simulink model "controllo_motori"  (R2025b)
settings: Solver=FixedStepAuto  StartTime=0.0  StopTime=10  FixedStep=0.01  RelTol=1e-3
libraries: slpidlib x3, vehdynlibtire x2, simulink x2, vehdynlibsteering x1, autolibshared x1
(part 1 of 2)
settings Model: SimulationMode=accelerator  Creator=lori2  LastModifiedBy=zinga

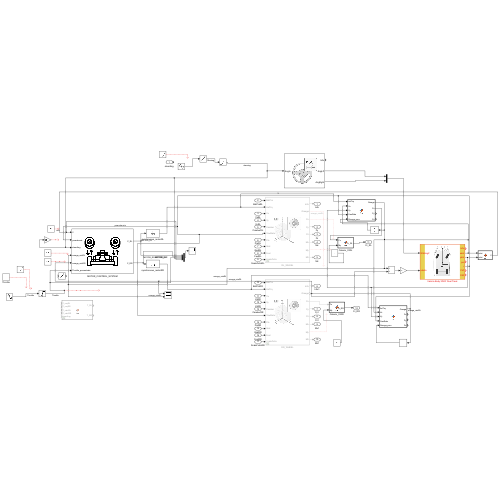
[thumbnail: Simulink's stored preview of the top-level diagram]
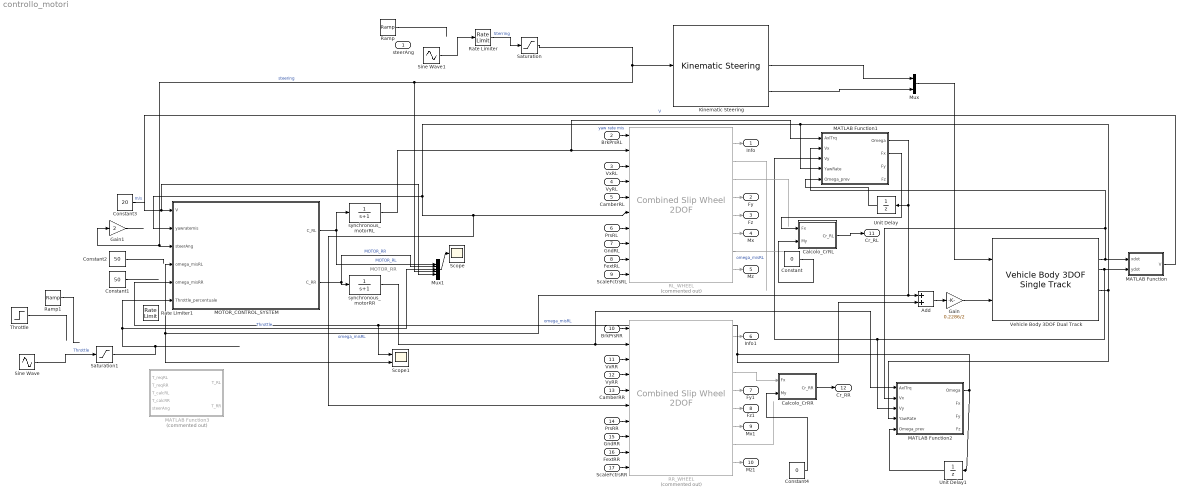
== system controllo_motori ==
  note: MOTOR_RR
  steerAng : Inport
  BrkPrsRL : Inport  Port=2
  VxRL : Inport  Port=3
  VyRL : Inport  Port=4
  CamberRL : Inport  Port=5
  PrsRL : Inport  Port=6
  GndRL : Inport  Port=7
  FextRL : Inport  Port=8
  ScaleFctrsRL : Inport  Port=9
  BrkPrsRR : Inport  Port=10
  VxRR : Inport  Port=11
  VyRR : Inport  Port=12
  CamberRR : Inport  Port=13
  PrsRR : Inport  Port=14
  GndRR : Inport  Port=15
  FextRR : Inport  Port=16
  ScaleFctrsRR : Inport  Port=17
  Add : Sum
  Calcolo_CrRL : MATLAB Function  TreatAsAtomicUnit=on
  Calcolo_CrRR : MATLAB Function  TreatAsAtomicUnit=on
  Constant : Constant  Value=0
  Constant1 : Constant  Value=50
  Constant2 : Constant  Value=50
  Constant3 : Constant  Value=20
  Constant4 : Constant  Value=0
  Gain : Gain  Gain=0.2286/2
  Gain1 : Gain  Gain=2
  Kinematic Steering : vehdynlibsteering/Kinematic Steering  StrgType=Ackerman  StrgRatioType=Constant  Loc=Front  NrmlFctr=0.01  TrckWdth=1.2  WhlBase=0.336  Db=0  StrgRng=1.25*pi  StrgAngBpts="[-6.2832   -5.0265   -3.7699   -2.5133   -1.2566         0    1.2566    2.5133    3.7699    5.0265    6.2832]"  StrgRatioTbl=|  StrgRatio=100  PctAckIn=off  PctAck=100  PctAckTbl=ones(1,11)*100  StrgArmLngth=0.1  RckCsLngth=0.5  TieRodLngth=0.248  D=0.2  PnnRadius=0.00085818  PnnRadiusTbl="[0.0055    0.0055    0.0056    0.0057    0.0058    0.0057    0.0057    0.0057    0.0056    0.0055    0.0055]"  RodLngth=0.1  ParaArmLngth=0.9  aMode=2
      | [13.5000   13.3750   13.2500   13.1250   13.0000   13.0000   13.0000   13.1250   13.2500   13.3750   13.5000
      | ]
  MATLAB Function : MATLAB Function  TreatAsAtomicUnit=on
  MATLAB Function1 : MATLAB Function  TreatAsAtomicUnit=on
  MATLAB Function2 : MATLAB Function  TreatAsAtomicUnit=on
  MATLAB Function3 : MATLAB Function  Commented=on  TreatAsAtomicUnit=on
  MOTOR_CONTROL_SYSTEM : Subsystem
      mask Display: image('car_16221049.png', [0,0,0,0,80,80]);
  Mux : Mux  Inputs=2
  Mux1 : Mux  Inputs=5
  RL_WHEEL : vehdynlibtire/Combined Slip Wheel 2DOF  Commented=on  tireType=External file  tireParamSet=vdynPassCar.mat  vertType=Magic Formula  plySteer=on  turnslip=on  BrakeType=Disc  mu_static=.3  mu_kinetic=.2  drum_abore=0.0508  drum_a=0.123  drum_c=0.212  drum_r=0.15  drum_theta1=0  drum_theta2=126  disk_abore=.05  Rm=.177  num_pads=2  brake_p_bpt=[1 11.4736842105263 21.9473684210526 32.4210526315789 42.8947368421053 53.3684210526316 63.8421052631579 74.3157894736842 84.7894736842105 95.2631578947368 105.736842105263 116.210526315789 126.684210526316 137.157894736842 147.631578947368 158.105263157895 168.578947368421 179.052631578947 189.526315789474 200]  brake_n_bpt=[0 52.6315789473684 105.263157894737 157.894736842105 210.526315789474 263.157894736842 315.789473684211 368.421052631579 421.052631578947 473.684210526316 526.315789473684 578.947368421053 631.578947368421 684.210526315789 736.842105263158 789.473684210526 842.105263157895 894.736842105263 947.368421052632 1000]  f_brake_t=[43.4900602404453 42.5056030554862 41.5350898940194 40.5780454442085 39.6340111501808 38.7025443887544 37.7832176914519 36.8756180088306 35.9793460143796 35.0940154454303 34.2192524787115 33.3546951383474 32.4999927342521 31.6548053290159 30.8188032315107 29.991666515561 29.1730845621415 28.362755623661 27.5603864089927 26.765691687993;498.991217495636 487.695866636631 476.560505099801 465.579679307235 454.748127933653 444.060772460445 433.51270824929 423.099196101319 412.81565427025 402.657650900201 392.620896861006 382.701238955775 372.894653477208 363.197240090814 353.605216024701 344.114910546964 334.722759712992 325.425301366216 316.219170376863 307.10109410434;954.492374750826 932.886130217776 911.585920305583 890.581313170261 869.862244717126 849.419000532136 829.242198807128 809.322774193808 789.651962526121 770.221286354971 751.0225412433 732.047782773203 713.289314220164 694.739674852612 676.391628817892 658.238154578366 640.272434863842 622.48784710877 604.877954344734 587.436496520688;1409.99353200602 1378.07639379892 1346.61133551136 1315.58294703329 1284.9763615006 1254.77722860383 1224.97168936497 1195.5463522863 1166.48827078199 1137.78492180974 1109.42418562559 1081.39432659063 1053.68397496312 1026.28210961441 999.178041611083 972.361398609768 945.822110014692 919.550392851325 893.536738312604 867.771898937035;1865.49468926121 1823.26665738007 1781.63675071715 1740.58458089631 1700.09047828407 1660.13545667552 1620.7011799228 1581.76993037878 1543.32457903786 1505.34855726451 1467.82583000789 1430.74087040806 1394.07863570608 1357.82454437621 1321.96445440427 1286.48464264117 1251.37178516554 1216.61293859388 1182.19552228048 1148.10730135338;2320.9958465164 2268.45692096121 2216.66216592293 2165.58621475934 2115.20459506754 2065.49368474721 2016.43067048064 1967.99350847127 1920.16088729373 1872.91219271928 1826.22747439018 1780.08741422549 1734.47329644903 1689.36697913801 1644.75086719747 1600.60788667257 1556.92146031639 1513.67548433643 1470.85430624835 1428.44270376973;2776.49700377159 2713.64718454235 2651.68758112871 2590.58784862237 2530.31871185102 2470.8519128189 2412.16016103848 2354.21708656376 2296.9971955496 2240.47582817405 2184.62911877248 2129.43395804292 2074.86795719199 2020.9094138998 1967.53727999066 1914.73113070398 1862.47113546724 1810.73803007899 1759.51309021622 1708.77810618608;3231.99816102678 3158.8374481235 3086.71299633449 3015.58948248539 2945.43282863449 2876.21014089059 2807.88965159632 2740.44066465625 2673.83350380547 2608.03946362882 2543.03076315477 2478.78050186034 2415.26261793494 2352.4518486616 2290.32369278385 2228.85437473538 2168.02081061809 2107.80057582154 2048.17187418409 1989.11350860242;3687.49931828197 3604.02771170464 3521.73841154027 3440.59111634842 3360.54694541796 3281.56836896228 3203.61914215416 3126.66424274874 3050.66981206134 2975.60309908359 2901.43240753707 2828.12704567777 2755.6572786779 2683.9942834234 2613.11010557704 2542.97761876678 2473.57048576894 2404.8631215641 2336.83065815196 2269.44891101877;4143.00047553716 4049.21797528579 3956.76382674606 3865.59275021144 3775.66106220143 3686.92659703397 3599.34863271199 3512.88782084123 3427.50612031721 3343.16673453836 3259.83405191936 3177.4735894952 3096.05193942085 3015.5367181852 2935.89651837023 2857.10086279818 2779.12016091979 2701.92566730665 2625.48944211983 2549.78431343512;4598.50163279235 4494.40823886693 4391.78924195184 4290.59438407447 4190.77517898491 4092.28482510566 3995.07812326983 3899.11139893372 3804.34242857308 3710.73036999313 3618.23569630166 3526.82013331263 3436.44660016381 3347.079152947 3258.68293116342 3171.22410682959 3084.66983607064 2998.98821304921 2914.1482260877 2830.11971585147;5054.00279004754 4939.59850244808 4826.81465715762 4715.59601793749 4605.88929576838 4497.64305317735 4390.80761382767 4285.3349770262 4181.17873682896 4078.2940054479 3976.63734068395 3876.16667713006 3776.84126090677 3678.62158770879 3581.46934395661 3485.34735086099 ...(+2764 chars)]  NOMPRES=262000  PRESMAX=1000000  PRESMIN=10000  FNOMIN=4300  FZMAX=8600  FZMIN=100  VXLOW=1  KPUMAX=1.5  KPUMIN=-1.5  ALPMAX=1.5  ALPMIN=-1.5  CAMMAX=0.17453  CAMMIN=-0.17453  LONGVL=16.7  FxRelFreqLwrLim=200*pi  FyRelFreqLwrLim=200*pi  MyRelFreqLwrLim=100*pi  omegao=0  UNLOADED_RADIUS=0.33454  WIDTH=0.235  RIM_RADIUS=0.2286  ASPECT_RATIO=0.45  MASS=11.2  IYY=1.084  br=1e-3  GRAVITY=-9.81  zo=0  zdoto=0  BREFF=8.25094594147963  DREFF=0.260468730454265  FREFF=0.0735298544471851  Q_RE0=1.00866439868088  Q_V1=0.000760413786224011  Q_V2=0.0463384792019201  Q_FZ1=0  Q_FZ2=15.6870832810226  Q_FZ3=0  Q_FCX=0.138643970247602  Q_FCY=0.10843499565426  Q_FCY2=-0.465763352339538  PFZ1=0.69958166705601  VERTICAL_STIFFNESS=207885.061134007  VERTICAL_DAMPING=500  BOTTOM_OFFST=0.00990653336182505  BOTTOM_STIFF=1999075.87051971  Q_CAM1=86.7791723017291  Q_CAM2=259.705254231766  Q_CAM3=0.510281667378416  Q_FYS1=-20769.4728880343  Q_FYS2=-59060.183485617  Q_FYS3=89271.8260126986  LONGITUDINAL_STIFFNESS=388714.175879854  LATERAL_STIFFNESS=157087.404633332  PCFX1=0.18539229191199  PCFX2=0  PCFX3=0  PCFY1=0.163183345037677  PCFY2=0  PCFY3=0.249094918231954  Q_RA1=0.675942571700787  Q_RA2=0.73800463546164  Q_RB1=1.04487486456705  Q_RB2=-1.191763806629  PCX1=1.58523057950359  PDX1=1.0239116238178  PDX2=-0.0842405110022724  PDX3=0  PEX1=0.110312777158455  PEX2=0.313468516038146  PEX3=0  PEX4=0.0016060905760045  PKX1=21.3872544684023  PKX2=14.0006541873175  PKX3=-0.405326109653452  PHX1=0.000212599305364818  PHX2=0.00115950515263055  PVX1=1.59236164471432e-05  PVX2=0.000104321112127671  PPX1=-0.349461321276586  PPX2=0.387840040616429  PPX3=-0.0969947336569324  PPX4=0.0632271859795801  RBX1=12.7633329850276  RBX2=9.5787123658471  RBX3=0  RCX1=1.02796280922059  REX1=-0.45202516851367  REX2=-0.47304886171176  RHX1=0.000233272373115809  QSX1=-0.00788307788961443  QSX2=0.954629515459396  QSX3=0.0155855777667025  QSX4=0.125904607142414  QSX5=1.01110069703963  QSX6=20.1938577118433  QSX7=0.310818120717083  QSX8=-0.0430823751139655  QSX9=0.636494404888216  QSX10=0.142438060591663  QSX11=0.346766530036373  QSX12=0  QSX13=0  QSX14=0  PPMX1=0  PCY1=1.34299950037631  PDY1=0.878267729082195  PDY2=-0.0644597923147385  PDY3=0  PEY1=-0.809776534470972  PEY2=-0.600180598867198  PEY3=0.0991732552633487  PEY4=-6.5577974035573  PEY5=0  PKY1=-15.5714726518315  PKY2=1.73126522291751  PKY3=0.365349873517229  PKY4=1.98176755955416  PKY5=0  PKY6=-0.884005199550313  PKY7=-0.237259727611847  PHY1=-0.00183370557235628  PHY2=0.00346401302716671  PVY1=-0.00675427560163264  PVY2=0.036379218103843  PVY3=-0.163543984089166  PVY4=-0.491003349625726  PPY1=-0.62059646553185  PPY2=-0.0647824842338686  PPY3=-0.164648843290686  PPY4=0.283193909060098  PPY5=0  RBY1=10.7588809173639  RBY2=7.70420065295029  RBY3=3.40283755070691e-06  RBY4=0  RCY1=1.06691874059059  REY1=0.308244924574305  REY2=7.48775032604508e-06  RHY1=0.0118479204960415  RHY2=7.63650177161071e-06  RVY1=0.0560024425050078  RVY2=7.48487127056197e-06  RVY3=0  RVY4=98.4047026517149  RVY5=2.02759273900054  RVY6=15.7623064923347  QSY1=0.00699077564863536  QSY2=0  QSY3=0.00153535478298811  QSY4=8.55710322455322e-05  QSY5=0  QSY6=0  QSY7=0.89443879773793  QSY8=-0.403227641260894  QBZ1=11.666656027484  QBZ2=-1.30355438574485  QBZ3=0  QBZ4=0.177918305399071  QBZ5=-0.162481135068033  QBZ6=0  QBZ9=30.1445534682089  QBZ10=0  QCZ1=1.29026978207574  QDZ1=0.0886972644991399  QDZ2=-0.0058634820161856  QDZ3=0.3805597481383  QDZ4=0  QDZ6=0.00160914918118959  QDZ7=-0.00211036330862154  QDZ8=-0.13921904912557  QDZ9=0.00816585550028243  QDZ10=0  QDZ11=0  QEZ1=-2.19802254534746  QEZ2=1.01850535789165  QEZ3=0  QEZ4=0.278379679112054  QEZ5=-0.548414722765386  QHZ1=0.00148361198869669  QHZ2=0.00202017567585904  QHZ3=0.240316641332066  QHZ4=-0.210114035738085  PPZ1=-0.443927982388615  PPZ2=0  SSZ1=0.00914999585397887  SSZ2=0.0389830656052735  SSZ3=0  SSZ4=0  PDXP1=0.396718274678791  PDXP2=0  PDXP3=0  PKYP1=1.00587060633573  PDYP1=0.40483048923438  PDYP2=0  PDYP3=0  PDYP4=0  PHYP1=0.992731942067188  PHYP2=0.150352945499914  PHYP3=0  PHYP4=-3.98988682633674  PECP1=0.502379254513503  PECP2=0  QDTP1=10.0178654287947  QCRP1=0.200627747200702  QCRP2=0.0995735881599772  QBRP1=0.0997107127960717  QDRP1=1.01432910167423  QDRP2=0  aMode=2
  RR_WHEEL : vehdynlibtire/Combined Slip Wheel 2DOF  Commented=on  tireType=External file  tireParamSet=vdynPassCar.mat  vertType=Magic Formula  plySteer=on  turnslip=on  BrakeType=Disc  mu_static=.3  mu_kinetic=.2  drum_abore=0.0508  drum_a=0.123  drum_c=0.212  drum_r=0.15  drum_theta1=0  drum_theta2=126  disk_abore=.05  Rm=.177  num_pads=2  brake_p_bpt=[1 11.4736842105263 21.9473684210526 32.4210526315789 42.8947368421053 53.3684210526316 63.8421052631579 74.3157894736842 84.7894736842105 95.2631578947368 105.736842105263 116.210526315789 126.684210526316 137.157894736842 147.631578947368 158.105263157895 168.578947368421 179.052631578947 189.526315789474 200]  brake_n_bpt=[0 52.6315789473684 105.263157894737 157.894736842105 210.526315789474 263.157894736842 315.789473684211 368.421052631579 421.052631578947 473.684210526316 526.315789473684 578.947368421053 631.578947368421 684.210526315789 736.842105263158 789.473684210526 842.105263157895 894.736842105263 947.368421052632 1000]  f_brake_t=[43.4900602404453 42.5056030554862 41.5350898940194 40.5780454442085 39.6340111501808 38.7025443887544 37.7832176914519 36.8756180088306 35.9793460143796 35.0940154454303 34.2192524787115 33.3546951383474 32.4999927342521 31.6548053290159 30.8188032315107 29.991666515561 29.1730845621415 28.362755623661 27.5603864089927 26.765691687993;498.991217495636 487.695866636631 476.560505099801 465.579679307235 454.748127933653 444.060772460445 433.51270824929 423.099196101319 412.81565427025 402.657650900201 392.620896861006 382.701238955775 372.894653477208 363.197240090814 353.605216024701 344.114910546964 334.722759712992 325.425301366216 316.219170376863 307.10109410434;954.492374750826 932.886130217776 911.585920305583 890.581313170261 869.862244717126 849.419000532136 829.242198807128 809.322774193808 789.651962526121 770.221286354971 751.0225412433 732.047782773203 713.289314220164 694.739674852612 676.391628817892 658.238154578366 640.272434863842 622.48784710877 604.877954344734 587.436496520688;1409.99353200602 1378.07639379892 1346.61133551136 1315.58294703329 1284.9763615006 1254.77722860383 1224.97168936497 1195.5463522863 1166.48827078199 1137.78492180974 1109.42418562559 1081.39432659063 1053.68397496312 1026.28210961441 999.178041611083 972.361398609768 945.822110014692 919.550392851325 893.536738312604 867.771898937035;1865.49468926121 1823.26665738007 1781.63675071715 1740.58458089631 1700.09047828407 1660.13545667552 1620.7011799228 1581.76993037878 1543.32457903786 1505.34855726451 1467.82583000789 1430.74087040806 1394.07863570608 1357.82454437621 1321.96445440427 1286.48464264117 1251.37178516554 1216.61293859388 1182.19552228048 1148.10730135338;2320.9958465164 2268.45692096121 2216.66216592293 2165.58621475934 2115.20459506754 2065.49368474721 2016.43067048064 1967.99350847127 1920.16088729373 1872.91219271928 1826.22747439018 1780.08741422549 1734.47329644903 1689.36697913801 1644.75086719747 1600.60788667257 1556.92146031639 1513.67548433643 1470.85430624835 1428.44270376973;2776.49700377159 2713.64718454235 2651.68758112871 2590.58784862237 2530.31871185102 2470.8519128189 2412.16016103848 2354.21708656376 2296.9971955496 2240.47582817405 2184.62911877248 2129.43395804292 2074.86795719199 2020.9094138998 1967.53727999066 1914.73113070398 1862.47113546724 1810.73803007899 1759.51309021622 1708.77810618608;3231.99816102678 3158.8374481235 3086.71299633449 3015.58948248539 2945.43282863449 2876.21014089059 2807.88965159632 2740.44066465625 2673.83350380547 2608.03946362882 2543.03076315477 2478.78050186034 2415.26261793494 2352.4518486616 2290.32369278385 2228.85437473538 2168.02081061809 2107.80057582154 2048.17187418409 1989.11350860242;3687.49931828197 3604.02771170464 3521.73841154027 3440.59111634842 3360.54694541796 3281.56836896228 3203.61914215416 3126.66424274874 3050.66981206134 2975.60309908359 2901.43240753707 2828.12704567777 2755.6572786779 2683.9942834234 2613.11010557704 2542.97761876678 2473.57048576894 2404.8631215641 2336.83065815196 2269.44891101877;4143.00047553716 4049.21797528579 3956.76382674606 3865.59275021144 3775.66106220143 3686.92659703397 3599.34863271199 3512.88782084123 3427.50612031721 3343.16673453836 3259.83405191936 3177.4735894952 3096.05193942085 3015.5367181852 2935.89651837023 2857.10086279818 2779.12016091979 2701.92566730665 2625.48944211983 2549.78431343512;4598.50163279235 4494.40823886693 4391.78924195184 4290.59438407447 4190.77517898491 4092.28482510566 3995.07812326983 3899.11139893372 3804.34242857308 3710.73036999313 3618.23569630166 3526.82013331263 3436.44660016381 3347.079152947 3258.68293116342 3171.22410682959 3084.66983607064 2998.98821304921 2914.1482260877 2830.11971585147;5054.00279004754 4939.59850244808 4826.81465715762 4715.59601793749 4605.88929576838 4497.64305317735 4390.80761382767 4285.3349770262 4181.17873682896 4078.2940054479 3976.63734068395 3876.16667713006 3776.84126090677 3678.62158770879 3581.46934395661 3485.34735086099 ...(+2764 chars)]  NOMPRES=262000  PRESMAX=1000000  PRESMIN=10000  FNOMIN=4300  FZMAX=8600  FZMIN=100  VXLOW=1  KPUMAX=1.5  KPUMIN=-1.5  ALPMAX=1.5  ALPMIN=-1.5  CAMMAX=0.17453  CAMMIN=-0.17453  LONGVL=16.7  FxRelFreqLwrLim=200*pi  FyRelFreqLwrLim=200*pi  MyRelFreqLwrLim=100*pi  omegao=0  UNLOADED_RADIUS=0.33454  WIDTH=0.235  RIM_RADIUS=0.2286  ASPECT_RATIO=0.45  MASS=11.2  IYY=1.084  br=1e-3  GRAVITY=-9.81  zo=0  zdoto=0  BREFF=8.25094594147963  DREFF=0.260468730454265  FREFF=0.0735298544471851  Q_RE0=1.00866439868088  Q_V1=0.000760413786224011  Q_V2=0.0463384792019201  Q_FZ1=0  Q_FZ2=15.6870832810226  Q_FZ3=0  Q_FCX=0.138643970247602  Q_FCY=0.10843499565426  Q_FCY2=-0.465763352339538  PFZ1=0.69958166705601  VERTICAL_STIFFNESS=207885.061134007  VERTICAL_DAMPING=500  BOTTOM_OFFST=0.00990653336182505  BOTTOM_STIFF=1999075.87051971  Q_CAM1=86.7791723017291  Q_CAM2=259.705254231766  Q_CAM3=0.510281667378416  Q_FYS1=-20769.4728880343  Q_FYS2=-59060.183485617  Q_FYS3=89271.8260126986  LONGITUDINAL_STIFFNESS=388714.175879854  LATERAL_STIFFNESS=157087.404633332  PCFX1=0.18539229191199  PCFX2=0  PCFX3=0  PCFY1=0.163183345037677  PCFY2=0  PCFY3=0.249094918231954  Q_RA1=0.675942571700787  Q_RA2=0.73800463546164  Q_RB1=1.04487486456705  Q_RB2=-1.191763806629  PCX1=1.58523057950359  PDX1=1.0239116238178  PDX2=-0.0842405110022724  PDX3=0  PEX1=0.110312777158455  PEX2=0.313468516038146  PEX3=0  PEX4=0.0016060905760045  PKX1=21.3872544684023  PKX2=14.0006541873175  PKX3=-0.405326109653452  PHX1=0.000212599305364818  PHX2=0.00115950515263055  PVX1=1.59236164471432e-05  PVX2=0.000104321112127671  PPX1=-0.349461321276586  PPX2=0.387840040616429  PPX3=-0.0969947336569324  PPX4=0.0632271859795801  RBX1=12.7633329850276  RBX2=9.5787123658471  RBX3=0  RCX1=1.02796280922059  REX1=-0.45202516851367  REX2=-0.47304886171176  RHX1=0.000233272373115809  QSX1=-0.00788307788961443  QSX2=0.954629515459396  QSX3=0.0155855777667025  QSX4=0.125904607142414  QSX5=1.01110069703963  QSX6=20.1938577118433  QSX7=0.310818120717083  QSX8=-0.0430823751139655  QSX9=0.636494404888216  QSX10=0.142438060591663  QSX11=0.346766530036373  QSX12=0  QSX13=0  QSX14=0  PPMX1=0  PCY1=1.34299950037631  PDY1=0.878267729082195  PDY2=-0.0644597923147385  PDY3=0  PEY1=-0.809776534470972  PEY2=-0.600180598867198  PEY3=0.0991732552633487  PEY4=-6.5577974035573  PEY5=0  PKY1=-15.5714726518315  PKY2=1.73126522291751  PKY3=0.365349873517229  PKY4=1.98176755955416  PKY5=0  PKY6=-0.884005199550313  PKY7=-0.237259727611847  PHY1=-0.00183370557235628  PHY2=0.00346401302716671  PVY1=-0.00675427560163264  PVY2=0.036379218103843  PVY3=-0.163543984089166  PVY4=-0.491003349625726  PPY1=-0.62059646553185  PPY2=-0.0647824842338686  PPY3=-0.164648843290686  PPY4=0.283193909060098  PPY5=0  RBY1=10.7588809173639  RBY2=7.70420065295029  RBY3=3.40283755070691e-06  RBY4=0  RCY1=1.06691874059059  REY1=0.308244924574305  REY2=7.48775032604508e-06  RHY1=0.0118479204960415  RHY2=7.63650177161071e-06  RVY1=0.0560024425050078  RVY2=7.48487127056197e-06  RVY3=0  RVY4=98.4047026517149  RVY5=2.02759273900054  RVY6=15.7623064923347  QSY1=0.00699077564863536  QSY2=0  QSY3=0.00153535478298811  QSY4=8.55710322455322e-05  QSY5=0  QSY6=0  QSY7=0.89443879773793  QSY8=-0.403227641260894  QBZ1=11.666656027484  QBZ2=-1.30355438574485  QBZ3=0  QBZ4=0.177918305399071  QBZ5=-0.162481135068033  QBZ6=0  QBZ9=30.1445534682089  QBZ10=0  QCZ1=1.29026978207574  QDZ1=0.0886972644991399  QDZ2=-0.0058634820161856  QDZ3=0.3805597481383  QDZ4=0  QDZ6=0.00160914918118959  QDZ7=-0.00211036330862154  QDZ8=-0.13921904912557  QDZ9=0.00816585550028243  QDZ10=0  QDZ11=0  QEZ1=-2.19802254534746  QEZ2=1.01850535789165  QEZ3=0  QEZ4=0.278379679112054  QEZ5=-0.548414722765386  QHZ1=0.00148361198869669  QHZ2=0.00202017567585904  QHZ3=0.240316641332066  QHZ4=-0.210114035738085  PPZ1=-0.443927982388615  PPZ2=0  SSZ1=0.00914999585397887  SSZ2=0.0389830656052735  SSZ3=0  SSZ4=0  PDXP1=0.396718274678791  PDXP2=0  PDXP3=0  PKYP1=1.00587060633573  PDYP1=0.40483048923438  PDYP2=0  PDYP3=0  PDYP4=0  PHYP1=0.992731942067188  PHYP2=0.150352945499914  PHYP3=0  PHYP4=-3.98988682633674  PECP1=0.502379254513503  PECP2=0  QDTP1=10.0178654287947  QCRP1=0.200627747200702  QCRP2=0.0995735881599772  QBRP1=0.0997107127960717  QDRP1=1.01432910167423  QDRP2=0  aMode=2
  Ramp : simulink/Sources/Ramp  slope=-20  start=3  InitialOutput=0
  Ramp1 : simulink/Sources/Ramp  slope=10  start=0  InitialOutput=0
  Rate Limiter : RateLimiter  RisingSlewLimit=20  FallingSlewLimit=-20  SampleTimeMode=inherited
  Rate Limiter1 : RateLimiter  RisingSlewLimit=50  SampleTimeMode=inherited
  Saturation : Saturate  UpperLimit=25  LowerLimit=-25
  Saturation1 : Saturate  UpperLimit=100  LowerLimit=0
  Scope : Scope
      settings: ActiveDisplayYMinimum=-40.624996036647921  ActiveDisplayYMaximum=115.62496432983133
  Scope1 : Scope  NumInputPorts=2
      settings: ActiveDisplayYMinimum=-33.400578421241562  ActiveDisplayYMaximum=300.60520579117411  DataLoggingVariableName=ScopeData2
  Sine Wave : Sin  Amplitude=100  Frequency=0.1  SampleTime=0.05
  Sine Wave1 : Sin  Amplitude=-30  Frequency=0.1  Phase=pi/4  SampleTime=0
  Throttle : Step  After=100  SampleTime=0
  Unit Delay : UnitDelay  SampleTime=-1  HasFrameUpgradeWarning=on
  Unit Delay1 : UnitDelay  SampleTime=-1  HasFrameUpgradeWarning=on
  Vehicle Body 3DOF Dual Track : autolibshared/Vehicle Body 3DOF Single Track  trackMode=Dual  inputMode=External longitudinal velocity  frontSteerMode=on  rearSteerMode=off  windMode=off  muMode=off  extFMode=off  extMMode=off  htchFMode=off  htchMMode=off  extXo=off  extpsio=off  extxdoto=off  extro=off  extYo=off  extTamb=off  extydoto=off  aMode=2  NF=2  NR=2  m=250  a=0.775  b=0.775  h=0.35  dh=1  hh=0.2  X_o=0  xdot_o=0  CalphaMode=off  sigmaMode=on  d=0  hl=0  w=[0.6,0.6]  Cy_f=12e3  Cy_r=11e3  sigma_f=.1  sigma_r=.1  alpha_f_brk=[-0.785, -0.628, -0.471, -0.314, -0.157, 0.000, 0.157, 0.314, 0.471, 0.628, 0.785]  Cy_f_data=[2000, 3000, 4000, 5500, 7000, 9000, 7000, 5500, 4000, 3000, 2000]  alpha_r_brk=[-0.785, -0.628, -0.471, -0.314, -0.157, 0.000, 0.157, 0.314, 0.471, 0.628, 0.785]  Cy_r_data=[2000, 3000, 4000, 5500, 7000, 9000, 7000, 5500, 4000, 3000, 2000]  Y_o=0  ydot_o=0  Izz=4000  psi_o=0  r_o=0  Af=2  Cd=.3  Cl=.1  Cpm=.1  beta_w=[0 0.01:0.01:0.3]  Cs=[0:0.03:0.9]  Cym=[0 1e-6:0.01:0.3]  Pabs=101325  Tair=273  g=9.81  mu=1  xdot_tol=.01  Fznom=2400  Fxtire_sat=7e4  Fytire_sat=7e4  longOff=0  latOff=0  vertOff=0  wrapAng=off
      settings: LibrarySourceBlock=vehdynlibeom/Vehicle Body 3DOF Dual Track
  synchronous_motorRL : TransferFcn  Denominator=[1 1]
  synchronous_motorRR : TransferFcn  Denominator=[1 1]
  Info : Outport
  Fy : Outport  Port=2
  Fz : Outport  Port=3
  Mx : Outport  Port=4
  Mz : Outport  Port=5
  Info1 : Outport  Port=6
  Fy1 : Outport  Port=7
  Fz1 : Outport  Port=8
  Mx1 : Outport  Port=9
  Mz1 : Outport  Port=10
  Cr_RL : Outport  Port=11
  Cr_RR : Outport  Port=12
  wires:
  Kinematic Steering/2 -> Mux/1
  Kinematic Steering/3 -> Mux/2
  Mux/1 -> Vehicle Body 3DOF Dual Track/1
  Rate Limiter/1 -> Saturation/1  "Sterring"
  Vehicle Body 3DOF Dual Track/2 -> MATLAB Function2/2(Vx), MATLAB Function1/2(Vx), MATLAB Function/1(xdot)
  Vehicle Body 3DOF Dual Track/3 -> MATLAB Function2/3(Vy), MATLAB Function1/3(Vy), MATLAB Function/2(ydot)
  MATLAB Function/1(V) -> Mux1/5, MOTOR_CONTROL_SYSTEM/1(V)  "V"
  Gain/1 -> Vehicle Body 3DOF Dual Track/2
  RR_WHEEL/5 -> Fz1/1
  RR_WHEEL/1 -> Info1/1
  RR_WHEEL/6 -> Mx1/1
  Vehicle Body 3DOF Dual Track/5 -> MATLAB Function1/4(YawRate), MOTOR_CONTROL_SYSTEM/2(yawratemis), RR_WHEEL/6, RL_WHEEL/6, MATLAB Function2/4(YawRate)  "yaw rate mis"
  RL_WHEEL/7 -> ?
  VxRL/1 -> RL_WHEEL/3
  FextRR/1 -> RR_WHEEL/9
  PrsRL/1 -> RL_WHEEL/7
  RR_WHEEL/4 -> Fy1/1
  RR_WHEEL/3 -> Calcolo_CrRR/1(Fx)
  GndRL/1 -> RL_WHEEL/8
  RL_WHEEL/1 -> Info/1
  VyRR/1 -> RR_WHEEL/4
  BrkPrsRR/1 -> RR_WHEEL/1
  VyRL/1 -> RL_WHEEL/4
  Add/1 -> Gain/1
  RL_WHEEL/3 -> ?
  RR_WHEEL/8 -> Mz1/1
  MATLAB Function1/1(Omega) -> MOTOR_CONTROL_SYSTEM/4(omega_misRL), Scope1/2, Add/1, Unit Delay/1  "omega_misRL"
  RR_WHEEL/7 -> ?
  ScaleFctrsRL/1 -> RL_WHEEL/10
  VxRR/1 -> RR_WHEEL/3
  RL_WHEEL/4 -> Fy/1
  GndRR/1 -> RR_WHEEL/8
  FextRL/1 -> RL_WHEEL/9
  RL_WHEEL/8 -> Mz/1
  CamberRR/1 -> RR_WHEEL/5
  CamberRL/1 -> RL_WHEEL/5
  ScaleFctrsRR/1 -> RR_WHEEL/10
  RL_WHEEL/5 -> Fz/1
  RL_WHEEL/6 -> Mx/1
  BrkPrsRL/1 -> RL_WHEEL/1
  PrsRR/1 -> RR_WHEEL/7
  Calcolo_CrRL/1(Cr_RL) -> Cr_RL/1
  Calcolo_CrRR/1(Cr_RR) -> Cr_RR/1
  MOTOR_CONTROL_SYSTEM/1(C_RL) -> synchronous_motorRL/1, Mux1/1  "MOTOR_RL"
  synchronous_motorRL/1 -> MATLAB Function1/1(AxlTrq), RL_WHEEL/2
  MOTOR_CONTROL_SYSTEM/2(C_RR) -> synchronous_motorRR/1, Mux1/2  "MOTOR_RR"
  synchronous_motorRR/1 -> MATLAB Function2/1(AxlTrq), RR_WHEEL/2
  Mux1/1 -> Scope/1
  Ramp/1 -> ?
  Sine Wave/1 -> Saturation1/1  "Throttle"
  Constant2/1 -> ?
  Constant1/1 -> ?
  Constant3/1 -> ?  "m/s"
  Saturation/1 -> Gain1/1, MOTOR_CONTROL_SYSTEM/3(steerAng), Mux1/4, Kinematic Steering/1  "steering"
  Sine Wave1/1 -> Rate Limiter/1
  Saturation1/1 -> MOTOR_CONTROL_SYSTEM/6(Throttle_percentuale), Mux1/3  "Throttle"
  Gain1/1 -> ?
  Throttle/1 -> ?
  Ramp1/1 -> ?
  Unit Delay/1 -> MATLAB Function1/5(Omega_prev)
  MATLAB Function1/2(Fx) -> Calcolo_CrRL/1(Fx)
  Constant/1 -> Calcolo_CrRL/2(My)
  Constant4/1 -> Calcolo_CrRR/2(My)
  MATLAB Function2/1(Omega) -> Add/2, Scope1/1, MOTOR_CONTROL_SYSTEM/5(omega_misRR), Unit Delay1/1  "omega_misRL"
  Unit Delay1/1 -> MATLAB Function2/5(Omega_prev)
  RL_WHEEL/2 -> ?  "omega_misRL"

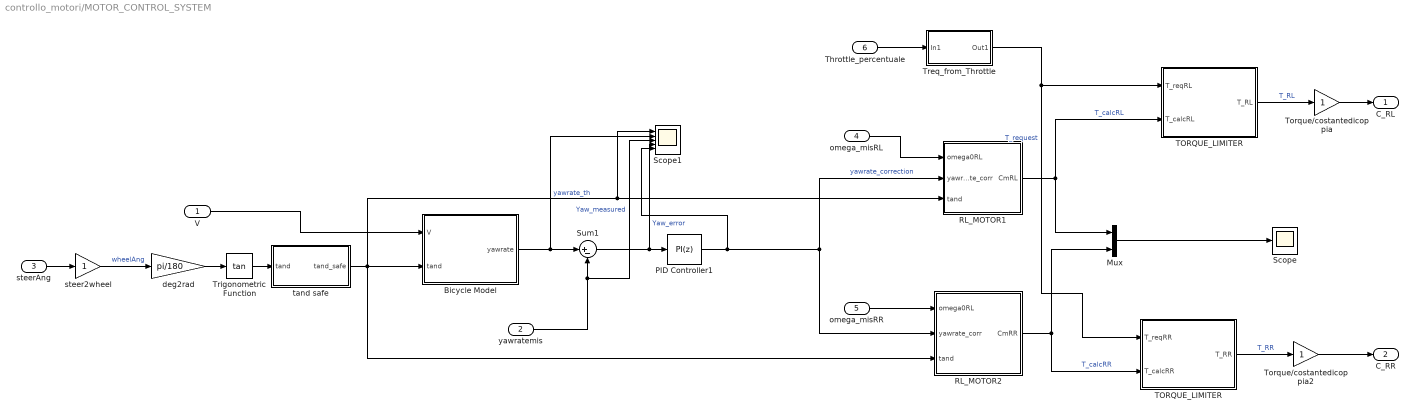
== system controllo_motori/MOTOR_CONTROL_SYSTEM ==
  V : Inport
  yawratemis : Inport  Port=2
  steerAng : Inport  Port=3
  omega_misRL : Inport  Port=4
  omega_misRR : Inport  Port=5
  Throttle_percentuale : Inport  Port=6
  " TORQUE_LIMITER" : MATLAB Function  TreatAsAtomicUnit=on
  Bicycle Model : MATLAB Function  TreatAsAtomicUnit=on
  Mux : Mux  Inputs=2
  PID Controller1 : slpidlib/PID Controller  Controller=PI  Form=Parallel  TimeDomain=Discrete-time  UseExternalTs=off  SampleTime=0.05  IntegratorMethod=Forward Euler  FilterMethod=Forward Euler  ControllerParametersSource=internal  P=0.6  I=0.005  UseKiTs=off  D=0  UseExternalDerivativeSource=off  N=100  UseFilter=on  TunerSelectOption=Transfer Function Based (PID Tuner App)  InitialConditionSource=internal  InitialConditionForIntegrator=0  InitialConditionForFilter=0  DifferentiatorICPrevScaledInput=0  ExternalReset=none  TrackingMode=off  Kt=1  LimitOutput=on  SatLimitsSource=internal  UpperSaturationLimit=5  LowerSaturationLimit=-5  LinearizeAsGain=on  AntiWindupMode=back-calculation  Kb=1  LimitIntegrator=off  UpperIntegratorSaturationLimit=inf  LowerIntegratorSaturationLimit=-inf  POutMin=[]  POutMax=[]  IOutMin=[]  IOutMax=[]  DOutMin=[]  DOutMax=[]  NOutMin=[]  NOutMax=[]  SumOutMin=[]  SumOutMax=[]  SaturationOutMin=[]  SaturationOutMax=[]  PParamMin=[]  PParamMax=[]  IParamMin=[]  IParamMax=[]  DParamMin=[]  DParamMax=[]  NParamMin=[]  NParamMax=[]  KbParamMin=[]  KbParamMax=[]  KtParamMin=[]  KtParamMax=[]  KbOutMin=[]  KbOutMax=[]  KtOutMin=[]  KtOutMax=[]  IntegratorOutMin=[]  IntegratorOutMax=[]  FilterOutMin=[]  FilterOutMax=[]  SumI1OutMin=[]  SumI1OutMax=[]  SumI2OutMin=[]  SumI2OutMax=[]  SumI3OutMin=[]  SumI3OutMax=[]  SumI4OutMin=[]  SumI4OutMax=[]  SumDOutMin=[]  SumDOutMax=[]  DifferentiatorOutMin=[]  DifferentiatorOutMax=[]  FilterDiffOutCoefMin=[]  FilterDiffOutCoefMax=[]  ReciprocalOutMin=[]  ReciprocalOutMax=[]  SumDenOutMin=[]  SumDenOutMax=[]  SumNumOutMin=[]  SumNumOutMax=[]  DivideOutMin=[]  DivideOutMax=[]  UdiffTsProdOutMin=[]  UdiffTsProdOutMax=[]  NTsProdOutMin=[]  NTsProdOutMax=[]  UintegralTsProdOutMin=[]  UintegralTsProdOutMax=[]  UngainTsProdOutMin=[]  UngainTsProdOutMax=[]  ClampingZeroOutDataTypeStr=Inherit: Inherit via back propagation  ClampingZeroOutMin=[]  ClampingZeroOutMax=[]  FilterDenConstantOutDataTypeStr=Inherit: Inherit via back propagation  FilterDenConstantOutMin=[]  FilterDenConstantOutMax=[]  PCopyOutDataTypeStr=Inherit: Inherit via back propagation  PCopyOutMin=[]  PCopyOutMax=[]  NCopyOutDataTypeStr=Inherit: Inherit via back propagation  NCopyOutMin=[]  NCopyOutMax=[]  IntegratorContinuousStateAttributes=''  IntegratorStateMustResolveToSignalObject=off  IntegratorRTWStateStorageClass=Auto  FilterContinuousStateAttributes=''  FilterStateMustResolveToSignalObject=off  FilterRTWStateStorageClass=Auto  ParallelPVariant=InternalParameters  IdealPVariant=Disabled  IVariant=InternalParameters  DVariant=Disabled  IntegratorVariant=Discrete  SatVariant=Enabled  AWVariant=BackCalculation  PCopyVariant=Disabled  TRVariant=Disabled  FdbkBlocksVariant=Forward  IdealPFdbkVariant=Disabled  SatFdbkVariant=Disabled  DerivativeFilterVariant=Disabled  NVariant=Disabled  NCopyVariant=Disabled_SignalSpec  FilterICVariant=Disabled  IntegratorICVariant=InternalICs  ExternalResetVariant=Disabled  TRSumVariant=Passthrough  SumFdbkVariant=Disabled  SumVariant=Sum_PI  TsampFilterVariant=InternalTs  TsampNgainVariant=Passthrough  TsampIntegralVariant=Disabled_SignalSpec  ExternalSaturationOutDataTypeStr=Inherit: Same as second input  DerivativeSourceVariant=Disabled  PreIntVariant=InternalPreInt
  RL_MOTOR1 : Subsystem
  RL_MOTOR2 : Subsystem
  Scope : Scope
      settings: ActiveDisplayYMinimum=-12.516207981515997  ActiveDisplayYMaximum=1.4170746352857368
  Scope1 : Scope  NumInputPorts=5
      settings: ActiveDisplayYMinimum=-4.4056435060424084  ActiveDisplayYMaximum=7.0392250929253359  DataLoggingVariableName=ScopeData4
  Sum1 : Sum  Inputs=|+-
  TORQUE_LIMITER : MATLAB Function  TreatAsAtomicUnit=on
  Torque/costantedicoppia : Gain
  Torque/costantedicoppia2 : Gain
  Treq_from_Throttle : Subsystem
  Trigonometric Function : Trigonometry  Operator=tan
  deg2rad : Gain  Gain=pi/180
  steer2wheel : Gain
  tand safe : MATLAB Function  TreatAsAtomicUnit=on
  C_RL : Outport
  C_RR : Outport  Port=2
  wires:
  PID Controller1/1 -> Scope1/5, RL_MOTOR2/2(yawrate_corr), RL_MOTOR1/2(yawrate_corr)  "yawrate_correction"
  Sum1/1 -> Scope1/4, PID Controller1/1  "Yaw_error"
  Bicycle Model/1(yawrate) -> Scope1/2, Sum1/1  "yawrate_th"
  tand safe/1(tand_safe) -> RL_MOTOR2/3(tand), RL_MOTOR1/3(tand), Scope1/1, Bicycle Model/2(tand)
  deg2rad/1 -> Trigonometric Function/1
  steerAng/1 -> steer2wheel/1
  yawratemis/1 -> Scope1/3, Sum1/2  "Yaw_measured"
  V/1 -> Bicycle Model/1(V)
  Torque/costantedicoppia2/1 -> C_RR/1
  omega_misRL/1 -> RL_MOTOR1/1(omega0RL)
  omega_misRR/1 -> RL_MOTOR2/1(omega0RL)
  RL_MOTOR1/1(CmRL) -> Mux/1, " TORQUE_LIMITER"/2(T_calcRL)  "T_calcRL"
  " TORQUE_LIMITER"/1(T_RL) -> Torque/costantedicoppia/1  "T_RL"
  RL_MOTOR2/1(CmRR) -> TORQUE_LIMITER/2(T_calcRR), Mux/2  "T_calcRR"
  TORQUE_LIMITER/1(T_RR) -> Torque/costantedicoppia2/1  "T_RR"
  Treq_from_Throttle/1(Out1) -> TORQUE_LIMITER/1(T_reqRR), " TORQUE_LIMITER"/1(T_reqRL)  "T_request"
  Throttle_percentuale/1 -> Treq_from_Throttle/1(In1)
  steer2wheel/1 -> deg2rad/1  "wheelAng"
  Mux/1 -> Scope/1
  Trigonometric Function/1 -> tand safe/1(tand)
  Torque/costantedicoppia/1 -> C_RL/1

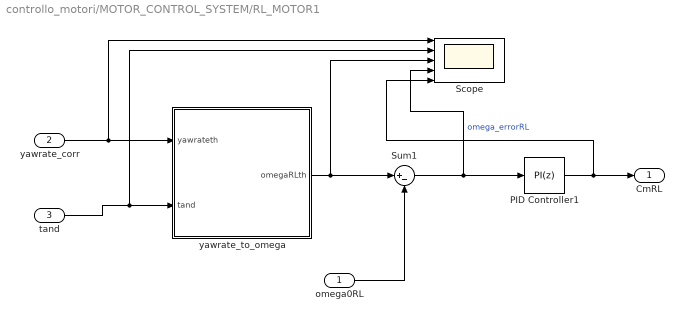
== system controllo_motori/MOTOR_CONTROL_SYSTEM/RL_MOTOR1 ==
  omega0RL : Inport
  yawrate_corr : Inport  Port=2
  tand : Inport  Port=3
  PID Controller1 : slpidlib/PID Controller  Controller=PI  Form=Parallel  TimeDomain=Discrete-time  UseExternalTs=off  SampleTime=0.03  IntegratorMethod=Forward Euler  FilterMethod=Forward Euler  ControllerParametersSource=internal  P=0.1  I=0  UseKiTs=off  D=0  UseExternalDerivativeSource=off  N=100  UseFilter=on  TunerSelectOption=Transfer Function Based (PID Tuner App)  InitialConditionSource=internal  InitialConditionForIntegrator=0  InitialConditionForFilter=0  DifferentiatorICPrevScaledInput=0  ExternalReset=none  TrackingMode=off  Kt=1  LimitOutput=on  SatLimitsSource=internal  UpperSaturationLimit=21  LowerSaturationLimit=-21  LinearizeAsGain=off  AntiWindupMode=clamping  Kb=1  LimitIntegrator=on  UpperIntegratorSaturationLimit=11  LowerIntegratorSaturationLimit=-11  POutMin=[]  POutMax=[]  IOutMin=[]  IOutMax=[]  DOutMin=[]  DOutMax=[]  NOutMin=[]  NOutMax=[]  SumOutMin=[]  SumOutMax=[]  SaturationOutMin=[]  SaturationOutMax=[]  PParamMin=[]  PParamMax=[]  IParamMin=[]  IParamMax=[]  DParamMin=[]  DParamMax=[]  NParamMin=[]  NParamMax=[]  KbParamMin=[]  KbParamMax=[]  KtParamMin=[]  KtParamMax=[]  KbOutMin=[]  KbOutMax=[]  KtOutMin=[]  KtOutMax=[]  IntegratorOutMin=[]  IntegratorOutMax=[]  FilterOutMin=[]  FilterOutMax=[]  SumI1OutMin=[]  SumI1OutMax=[]  SumI2OutMin=[]  SumI2OutMax=[]  SumI3OutMin=[]  SumI3OutMax=[]  SumI4OutMin=[]  SumI4OutMax=[]  SumDOutMin=[]  SumDOutMax=[]  DifferentiatorOutMin=[]  DifferentiatorOutMax=[]  FilterDiffOutCoefMin=[]  FilterDiffOutCoefMax=[]  ReciprocalOutMin=[]  ReciprocalOutMax=[]  SumDenOutMin=[]  SumDenOutMax=[]  SumNumOutMin=[]  SumNumOutMax=[]  DivideOutMin=[]  DivideOutMax=[]  UdiffTsProdOutMin=[]  UdiffTsProdOutMax=[]  NTsProdOutMin=[]  NTsProdOutMax=[]  UintegralTsProdOutMin=[]  UintegralTsProdOutMax=[]  UngainTsProdOutMin=[]  UngainTsProdOutMax=[]  ClampingZeroOutDataTypeStr=Inherit: Inherit via back propagation  ClampingZeroOutMin=[]  ClampingZeroOutMax=[]  FilterDenConstantOutDataTypeStr=Inherit: Inherit via back propagation  FilterDenConstantOutMin=[]  FilterDenConstantOutMax=[]  PCopyOutDataTypeStr=Inherit: Inherit via back propagation  PCopyOutMin=[]  PCopyOutMax=[]  NCopyOutDataTypeStr=Inherit: Inherit via back propagation  NCopyOutMin=[]  NCopyOutMax=[]  IntegratorContinuousStateAttributes=''  IntegratorStateMustResolveToSignalObject=off  IntegratorRTWStateStorageClass=Auto  FilterContinuousStateAttributes=''  FilterStateMustResolveToSignalObject=off  FilterRTWStateStorageClass=Auto  ParallelPVariant=InternalParameters  IdealPVariant=Disabled  IVariant=InternalParameters  DVariant=Disabled  IntegratorVariant=Discrete  SatVariant=Enabled  AWVariant=DiscClampingParallel  PCopyVariant=Disabled  TRVariant=Disabled  FdbkBlocksVariant=Forward  IdealPFdbkVariant=Disabled  SatFdbkVariant=Disabled  DerivativeFilterVariant=Disabled  NVariant=Disabled  NCopyVariant=Disabled_SignalSpec  FilterICVariant=Disabled  IntegratorICVariant=InternalICs  ExternalResetVariant=Disabled  TRSumVariant=Passthrough  SumFdbkVariant=Disabled  SumVariant=Sum_PI  TsampFilterVariant=InternalTs  TsampNgainVariant=Passthrough  TsampIntegralVariant=Disabled_SignalSpec  ExternalSaturationOutDataTypeStr=Inherit: Same as second input  DerivativeSourceVariant=Disabled  PreIntVariant=InternalPreInt
  Scope : Scope  NumInputPorts=5
      settings: ActiveDisplayYMinimum=-23.381836661538486  ActiveDisplayYMaximum=2.5979818512820536  DataLoggingVariableName=ScopeData3
  Sum1 : Sum  Inputs=|+-
  yawrate_to_omega : MATLAB Function  TreatAsAtomicUnit=on
  CmRL : Outport
  wires:
  Sum1/1 -> Scope/4, PID Controller1/1  "omega_errorRL"
  yawrate_corr/1 -> Scope/1, yawrate_to_omega/1(yawrateth)
  omega0RL/1 -> Sum1/2
  PID Controller1/1 -> Scope/5, CmRL/1
  yawrate_to_omega/1(omegaRLth) -> Scope/3, Sum1/1
  tand/1 -> Scope/2, yawrate_to_omega/2(tand)

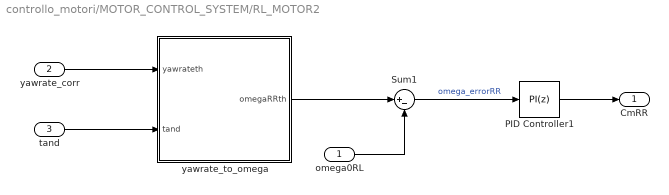
== system controllo_motori/MOTOR_CONTROL_SYSTEM/RL_MOTOR2 ==
  omega0RL : Inport
  yawrate_corr : Inport  Port=2
  tand : Inport  Port=3
  PID Controller1 : slpidlib/PID Controller  Controller=PI  Form=Parallel  TimeDomain=Discrete-time  UseExternalTs=off  SampleTime=0.03  IntegratorMethod=Forward Euler  FilterMethod=Forward Euler  ControllerParametersSource=internal  P=0.1  I=0  UseKiTs=on  D=0  UseExternalDerivativeSource=off  N=100  UseFilter=on  TunerSelectOption=Transfer Function Based (PID Tuner App)  InitialConditionSource=internal  InitialConditionForIntegrator=0  InitialConditionForFilter=0  DifferentiatorICPrevScaledInput=0  ExternalReset=none  TrackingMode=off  Kt=1  LimitOutput=on  SatLimitsSource=internal  UpperSaturationLimit=21  LowerSaturationLimit=-21  LinearizeAsGain=on  AntiWindupMode=clamping  Kb=1  LimitIntegrator=on  UpperIntegratorSaturationLimit=11  LowerIntegratorSaturationLimit=-11  POutMin=[]  POutMax=[]  IOutMin=[]  IOutMax=[]  DOutMin=[]  DOutMax=[]  NOutMin=[]  NOutMax=[]  SumOutMin=[]  SumOutMax=[]  SaturationOutMin=[]  SaturationOutMax=[]  PParamMin=[]  PParamMax=[]  IParamMin=[]  IParamMax=[]  DParamMin=[]  DParamMax=[]  NParamMin=[]  NParamMax=[]  KbParamMin=[]  KbParamMax=[]  KtParamMin=[]  KtParamMax=[]  KbOutMin=[]  KbOutMax=[]  KtOutMin=[]  KtOutMax=[]  IntegratorOutMin=[]  IntegratorOutMax=[]  FilterOutMin=[]  FilterOutMax=[]  SumI1OutMin=[]  SumI1OutMax=[]  SumI2OutMin=[]  SumI2OutMax=[]  SumI3OutMin=[]  SumI3OutMax=[]  SumI4OutMin=[]  SumI4OutMax=[]  SumDOutMin=[]  SumDOutMax=[]  DifferentiatorOutMin=[]  DifferentiatorOutMax=[]  FilterDiffOutCoefMin=[]  FilterDiffOutCoefMax=[]  ReciprocalOutMin=[]  ReciprocalOutMax=[]  SumDenOutMin=[]  SumDenOutMax=[]  SumNumOutMin=[]  SumNumOutMax=[]  DivideOutMin=[]  DivideOutMax=[]  UdiffTsProdOutMin=[]  UdiffTsProdOutMax=[]  NTsProdOutMin=[]  NTsProdOutMax=[]  UintegralTsProdOutMin=[]  UintegralTsProdOutMax=[]  UngainTsProdOutMin=[]  UngainTsProdOutMax=[]  ClampingZeroOutDataTypeStr=Inherit: Inherit via back propagation  ClampingZeroOutMin=[]  ClampingZeroOutMax=[]  FilterDenConstantOutDataTypeStr=Inherit: Inherit via back propagation  FilterDenConstantOutMin=[]  FilterDenConstantOutMax=[]  PCopyOutDataTypeStr=Inherit: Inherit via back propagation  PCopyOutMin=[]  PCopyOutMax=[]  NCopyOutDataTypeStr=Inherit: Inherit via back propagation  NCopyOutMin=[]  NCopyOutMax=[]  IntegratorContinuousStateAttributes=''  IntegratorStateMustResolveToSignalObject=off  IntegratorRTWStateStorageClass=Auto  FilterContinuousStateAttributes=''  FilterStateMustResolveToSignalObject=off  FilterRTWStateStorageClass=Auto  ParallelPVariant=InternalParameters  IdealPVariant=Disabled  IVariant=InternalParameters  DVariant=Disabled  IntegratorVariant=Discrete  SatVariant=Enabled  AWVariant=DiscClampingParallel  PCopyVariant=Disabled  TRVariant=Disabled  FdbkBlocksVariant=Forward  IdealPFdbkVariant=Disabled  SatFdbkVariant=Disabled  DerivativeFilterVariant=Disabled  NVariant=Disabled  NCopyVariant=Disabled_SignalSpec  FilterICVariant=Disabled  IntegratorICVariant=InternalICs  ExternalResetVariant=Disabled  TRSumVariant=Passthrough  SumFdbkVariant=Disabled  SumVariant=Sum_PI  TsampFilterVariant=InternalTs  TsampNgainVariant=Passthrough  TsampIntegralVariant=Disabled_SignalSpec  ExternalSaturationOutDataTypeStr=Inherit: Same as second input  DerivativeSourceVariant=Disabled  PreIntVariant=InternalPreInt
  Sum1 : Sum  Inputs=|+-
  yawrate_to_omega : MATLAB Function  TreatAsAtomicUnit=on
  CmRR : Outport
  wires:
  Sum1/1 -> PID Controller1/1  "omega_errorRR"
  yawrate_corr/1 -> yawrate_to_omega/1(yawrateth)
  omega0RL/1 -> Sum1/2
  PID Controller1/1 -> CmRR/1
  yawrate_to_omega/1(omegaRRth) -> Sum1/1
  tand/1 -> yawrate_to_omega/2(tand)

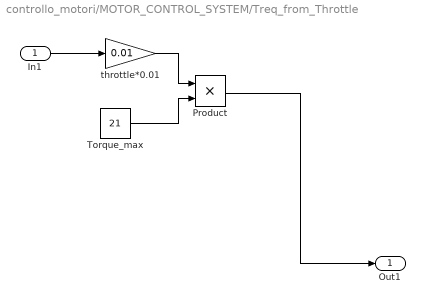
== system controllo_motori/MOTOR_CONTROL_SYSTEM/Treq_from_Throttle ==
  In1 : Inport
  Product : Product
  Torque_max : Constant  Value=21
  throttle*0.01 : Gain  Gain=0.01
  Out1 : Outport
  wires:
  throttle*0.01/1 -> Product/1
  In1/1 -> throttle*0.01/1
  Torque_max/1 -> Product/2
  Product/1 -> Out1/1

== matlab function controllo_motori/MATLAB Function2 ==
  data: AxlTrq input; Omega output; Vx input; Vy input; YawRate input; Omega_prev input; Fx output; Fy output; Fz output
function [Omega, Fx, Fy, Fz] = fcn(AxlTrq, Vx, Vy, YawRate, Omega_prev)
    % Parametri
    J   = 0.5;      % inerzia ruota+motore ridotta [kg·m²]
    Rw  = 0.2;      % raggio ruota [m]
    tau = 14.5;     % rapporto riduzione
    Cy  = 12000;    % rigidezza laterale pneumatico [N/rad]
    Ts  = 0.001;    % passo di integrazione [s]
    
    % Omega ruota (integrazione Eulero)
    alpha_ruota = AxlTrq / J;
    Omega = Omega_prev + alpha_ruota * Ts;
    Omega = max(0, Omega);  % no velocità negativa
    
    % Forza longitudinale
    Fx = AxlTrq * tau / Rw;
    
    % Angolo di deriva e forza laterale
    if abs(Vx) > 0.5
        slip_angle = atan2(Vy, abs(Vx)) - atan2(YawRate * 0.6, abs(Vx));
    else
        slip_angle = 0;
    end
    Fy = -Cy * slip_angle;
    
    % Forza verticale statica (peso per ruota)
    Fz = 280 * 9.81 / 4;   % [N]
end

== matlab function controllo_motori/MATLAB Function ==
  data: xdot input; V output; ydot input
function V = fcn(xdot,ydot)

V=(xdot^2 + ydot^2)^0.5;

== matlab function controllo_motori/MOTOR_CONTROL_SYSTEM/Bicycle Model ==
  data: V input; yawrate output; tand input
function yawrate = fcn(V, tand)
%#codegen
L = 1.55;  % passo del veicolo
yawrate = (V / L) * tand;

== matlab function controllo_motori/Calcolo_CrRL ==
  data: Fx input; Cr_RL output; My input
function Cr_RL = fcn(Fx,My)
R=0.3; % raggio ruota

Cr_RL=My + (Fx*R);

== matlab function controllo_motori/Calcolo_CrRR ==
  data: Fx input; Cr_RR output; My input
function Cr_RR = fcn(Fx,My)

R=0.3; % raggio ruota

Cr_RR=My + (Fx*R);

== matlab function controllo_motori/MOTOR_CONTROL_SYSTEM/ TORQUE_LIMITER ==
  data: T_reqRL input; T_RL output; T_calcRL input
function T_RL = fcn(T_reqRL, T_calcRL)
enable = T_reqRL > 0;  % 0 o 1

T_max = 21;
T_RL = max(0, min(T_max, T_reqRL + T_calcRL * enable));


% function T_RL = fcn(T_reqRL, T_calcRL)
%     T_max  = 21;
%     T_base = T_reqRL / 2;
%     T_RL   = max(0, min(T_max, T_base - T_calcRL));  
% end

== matlab function controllo_motori/MOTOR_CONTROL_SYSTEM/TORQUE_LIMITER ==
  data: T_reqRR input; T_RR output; T_calcRR input

function T_RR = fcn(T_reqRR, T_calcRR)
T_max = 21;
enable = T_reqRR > 0;  % 0 o 1

T_RR = max(0, min(T_max, T_reqRR - T_calcRR*enable));


% function T_RR = fcn(T_reqRR, T_calcRR)
%     T_max  = 21;
%     T_base = T_reqRR / 2;
%     T_RR   = max(0, min(T_max, T_base + T_calcRR));  
% end

== matlab function controllo_motori/MOTOR_CONTROL_SYSTEM/RL_MOTOR1/yawrate_to_omega ==
  data: yawrateth input; omegaRLth output; tand input
function omegaRLth = fcn(yawrateth,tand)

L=1.55; % passo veicolo
w = 1.2; % carreggiata veicolo
tau = 14.5; % rapporto di riduzione

% protezione divisione per zero
if abs(tand) < 0.01  % ~0.6 gradi, sotto questa soglia non agisce il TV
    omegaRLth = 0;
    return;
end

Rcg= ((L/2)^2 + (L/tand)^2)^0.5 ;  % raggio curvatura centro di massa
Rw=0.2; % raggio ruota
Rrl = L / tand; % raggio di curvatura ruota sinistra

gainRL=(tau / (Rcg * Rw * Rrl * L * tand));

omegaRLth=gainRL*yawrateth;

== matlab function controllo_motori/MOTOR_CONTROL_SYSTEM/RL_MOTOR2/yawrate_to_omega ==
  data: yawrateth input; omegaRRth output; tand input
function omegaRRth = fcn(yawrateth,tand)

L=1.55; % passo veicolo
w = 1.2; % carreggiata veicolo
tau = 14.5; % rapporto di riduzione

% protezione divisione per zero
if abs(tand) < 0.01  % ~0.6 gradi, sotto questa soglia non agisce il TV
    omegaRRth = 0;
    return;
end

Rcg= ((L/2)^2 + (L/tand)^2)^0.5 ;  % raggio curvatura centro di massa
Rw=0.2; % raggio ruota
Rrr = L / tand + w; % raggio di curvatura ruota destra

gainRR=(tau/(Rcg*Rw*Rrr*L*tand));

omegaRRth=gainRR*yawrateth;

== matlab function controllo_motori/MOTOR_CONTROL_SYSTEM/tand safe ==
  data: tand input; tand_safe output
% function tand_safe = fcn(tand)
%     tand_safe = sign(tand) * max(abs(tand), tan(2*pi/180));
% end

function tand_safe = fcn(tand)
    soglia = tan(5*pi/180);  % 5° invece di 2°
    
    if abs(tand) < soglia
        tand_safe = 0;  % TV disattivato sotto soglia
    else
        tand_safe = tand;  % passa il valore reale senza clamp
    end
end
